simulink model "UAclient"  (R2019b)
settings: Solver=ode1  StartTime=0.0  StopTime=70  FixedStep=0.001  RelTol=1e-3
undefined symbols (not defined in the file or in its folder): sigbuilder_block
settings Model: Creator=y0n  LastModifiedBy=y0n
settings DataIOCC: SaveOutput=off  SignalLogging=off  DSMLogging=off  SaveTime=off  ReturnWorkspaceOutputsName=VehicleOut
settings DebuggingCC: AlgebraicLoopMsg=none  UnderSpecifiedDimensionMsg=error
settings SFSimCC: CustomCodeUndefinedFunction=UseInterfaceOnly

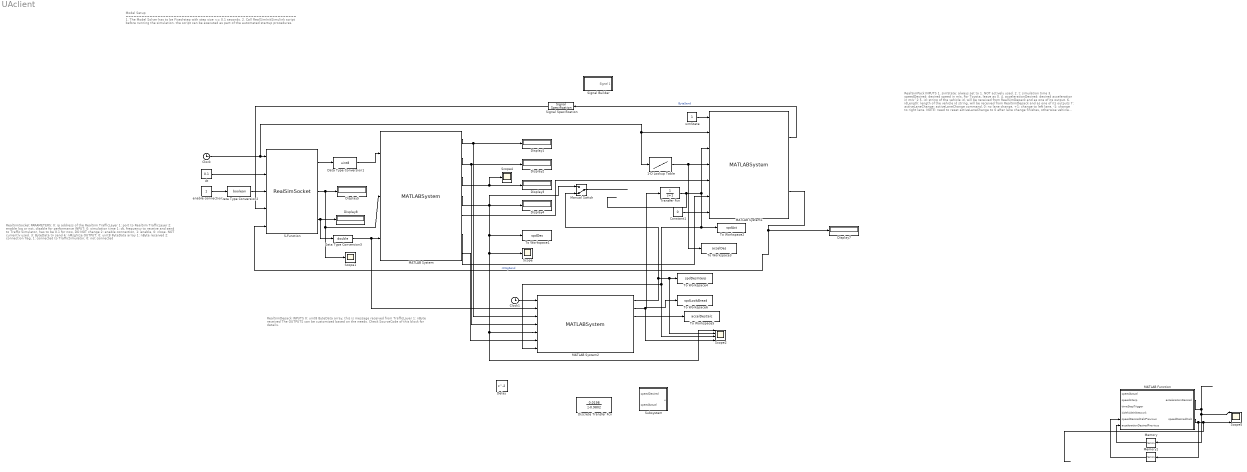
== system UAclient ==
  note: Model Setup
      | ================================================================
      | 1. The Model Solver has to be Fixed-step with step size <= 0.1 seconds.
      | 2. Call RealSimInitSimulink script before running the simulation. the script can be executed as part of the automated startup procedures.
  note: RealSimSocket
      | PARAMETERS:
      | 0: ip address of the RealSim TrafficLayer
      | 1: port to RealSim TrafficLayer
      | 2: enable log or not, disable for performance
      | INPUT:
      | 0: simulation time
      | 1: dt, frequency to receive and send to Traffic Simulator, has to be 0.1 for now, DO NOT change
      | 2: enable connection, 1: enable, 0: close. NOT currently used.
      | 3: ByteData to send
      | 4: nMsgSize
      |
      | OUTPUT:
      | 0: uint8 ByteData array
      | 1: nByte received
      | 2: connection flag, 1: connected to TrafficSimulator, 0: not connected
  note: RealSimPack
      | INPUTS
      | 1. simState: always set to 1. NOT actively used.
      | 2. t: simulation time
      | 3. speedDesired: desired speed in m/s, For Toyota, leave as 0.
      | 4. accelerationDesired: desired acceleration in m/s^2
      | 5. id: string of the vehicle id, will be received from RealSimDepack and as one of its output.
      | 6. idLength: length of the vehicle id string, will be received from RealSimDepack and as one of its outputs
      | 7: activeLaneChange: activeLaneChange command, 0: no lane change, +1: change to left lane, -1: change to right lane. NOTE: need to reset activeLaneChange to 0 after lane change finishes, otherwise vehicle will keep making lane change. Will receive 0 activeLaneChangeFdbk from RealSimDepack when lane change finishes.
      |
      | NOTE 1: Currently, only speedDesired and/or accelerationDesired can be sent to VISSIM/SUMO. The data format receive and send are the same so other mesage fields of the send data are irrelevant and can be set to empty or zero.
      |
      | NOTE 2: if select both speedDesired and accelerationDesired
      | in config.yaml, then only accelerationDesired will be used
      | to control vehicles in TrafficSimulator. if only one of
      | speedDesired and accelerationDesired selected in
      | config.yaml, then the one selected will be used for
      | control, the other input can be leave as 0.
      |
      | NOTE 3: for VISSIM, speedDesired or accelerationDesired will be the control command 0.2 seconds in the future.
      |
      | OUTPUTS
      | 1.ByteData: bytes vector that will be sent to TrafficSimualtor
      | 2.nMsgSize: size of bytes to be sent
  note: RealSimDepack
      | INPUTS
      | 0: uint8 ByteData array, this is message received from TrafficLayer
      | 1: nByte received
      |
      | The OUTPUTS can be customized based on the needs. Check SourceCode of this block for details.
  1-D Lookup Table : Lookup_n-D  NumberOfTableDimensions=1  BreakpointsForDimension1=[0 20 20.001 30 40 50 60 70 80 90 100]  Table=[0 0 0.2 0.2 -0.2 0.1 -0.1 0.3 -0.3 0 0 ]  InternalRulePriority=Speed  RndMeth=Simplest  InputSameDT=on
  Clock : Clock
  Clock1 : Clock
  Constant1 : Constant  Value=0
  Data Type Conversion1 : DataTypeConversion  OutDataTypeStr=uint8
  Data Type Conversion2 : DataTypeConversion  OutDataTypeStr=boolean
  Data Type Conversion3 : DataTypeConversion  OutDataTypeStr=double
  Delay : Delay
  Discrete Transfer Fcn : DiscreteTransferFcn  Numerator=[0.0198]  Denominator=[1 -0.9802]
  Display{1..5,7..8} (7 alike) : Display
  MATLAB Function : MATLAB Function  TreatAsAtomicUnit=on
  MATLAB System : MATLABSystem  System=RealSimDepack  VehicleMessageFieldDefInputVec=VehicleMessageFieldDefInputVec  SimulateUsing=Code generation
      mask Type: RealSimDepack
      mask Display:
      | disp('RealSimDepack');
      | port_label('input',1,'ByteData');
      | port_label('input',2,'nByte');
      | port_label('input',3,'connectionState');
      | port_label('output',1,'simState');
      | port_label('output',2,'t');
      | port_label('output',3,'nVeh');
      | port_label('output',4,'speed');
      | port_label('output',5,'id');
      | port_label('output',6,'idLen');
      | port_label('output',7,'isVehicleInNetwork');
  MATLAB System1 : MATLABSystem  System=RealSimPack  VehicleMessageFieldDefInputVec=VehicleMessageFieldDefInputVec  SimulateUsing=Code generation
      mask Type: RealSimPack
      mask Display:
      | disp('RealSimPack');
      | port_label('input',1,'simState');
      | port_label('input',2,'t');
      | port_label('input',3,'speedDesired');
      | port_label('input',4,'accelerationDesired');
      | port_label('input',5,'id');
      | port_label('input',6,'idLength');
      | port_label('input',7,'activeLaneChange');
      | port_label('output',1,'ByteData');
      | port_label('output',2,'nMsgSize');
  MATLAB System2 : MATLABSystem  System=RealSimInterpSpeed  initialSpeed=15.7  speedInterpolationMode=0  speedLookAheadHorizon=1  speedUpperBound=20  SimulateUsing=Code generation
      mask Type: RealSimInterpSpeed
      mask Display:
      | disp('RealSimInterpSpeed');
      | port_label('input',1,'simulationTime');
      | port_label('input',2,'connectionState');
      | port_label('input',3,'simState');
      | port_label('input',4,'timeReceive');
      | port_label('input',5,'speedReceive');
      | port_label('input',6,'isVehicleInNetwork');
      | port_label('input',7,'speedActual');
      | port_label('output',1,'speedInterp');
      | port_label('output',2,'speedLookAhead');
      | port_label('output',3,'accelerationDesired');
      | port_label('output',4,'timeSimulator');
      | port_label('output',5,'timeStepSimulator');
      | port_label('output',6,'timeStepTrigger');
      | port_label('output',7,'RealSimDelay');
  Manual Switch : ManualSwitch  CurrentSetting=0
  Memory : Memory
  Memory1 : Memory
  S-Function : S-Function  FunctionName=RealSimSocket  Parameters='127.0.0.1', 2333, 0  SFunctionDeploymentMode=off  EnableBusSupport=off
  Scope : Scope
  Scope1 : Scope
  Scope2 : Scope  NumInputPorts=4
  Scope4 : Scope
  Scope5 : Scope  NumInputPorts=4
  Signal Builder : Subsystem  Tag=STV Subsys  LoadFcn=sigbuilder_block('load');  StartFcn=sigbuilder_block('start');  StopFcn=sigbuilder_block('stop');  ClipboardFcn=sigbuilder_block('clipboard');  mask(Sigbuilder block){tuvar=[0:10]}
      mask help: Simulink:masks:SigbuilderBlock_MD
      mask init:
      | if ~strcmp(get_param(bdroot(gcbh),'SimulationStatus'),'stopped') tuvar = sigbuilder_block('maskInit'); end
      settings: CopyFcn=sigbuilder_block('copy');  DeleteFcn=sigbuilder_block('delete');  ModelCloseFcn=sigbuilder_block('modelClose');  PreSaveFcn=sigbuilder_block('preSave');  PauseFcn=sigbuilder_block('pause');  ContinueFcn=sigbuilder_block('continue');  NameChangeFcn=sigbuilder_block('namechange');  OpenFcn=sigbuilder_block('open',[6 30 1428 771.75 ]);  CloseFcn=sigbuilder_block('close');
      mask Display: plot(0, 0, 100, 100,[2, 2, 32, 32, 2], [68, 8, 8, 68, 68],[32, 2], [38, 38], [32, 19, 2],[53, 60, 44], [32, 17, 17, 2],[16, 16, 31, 31]);txt = getActiveGroup(gcbh);text(2, 100, txt,'verticalAlignment', 'top');
  Signal Specification : SignalSpecification  Dimensions=[200 1]
  Subsystem : Subsystem
  To Workspace1 : ToWorkspace  VariableName=spdDes  SaveFormat=Structure With Time  SampleTime=-1
  To Workspace2 : ToWorkspace  VariableName=spdAct  SaveFormat=Structure With Time  SampleTime=-1
  To Workspace3 : ToWorkspace  VariableName=accelDes  SaveFormat=Structure With Time  SampleTime=-1
  To Workspace4 : ToWorkspace  VariableName=spdDesInterp  SaveFormat=Structure With Time  SampleTime=-1
  To Workspace5 : ToWorkspace  VariableName=accelDesCalc  SaveFormat=Structure With Time  SampleTime=-1
  To Workspace6 : ToWorkspace  VariableName=spdLookAhead  SaveFormat=Structure With Time  SampleTime=-1
  Transfer Fcn : TransferFcn  Denominator=[1 1]
  dt : Constant  Value=0.1
  enable connection : Constant
  simState : Constant
  wires:
  Clock/1 -> MATLAB System1/2, 1-D Lookup Table/1, S-Function/1
  dt/1 -> S-Function/2
  simState/1 -> MATLAB System1/1
  MATLAB System1/1 -> Signal Specification/1  "ByteSend"
  MATLAB System1/2 -> S-Function/5, Display7/1  "nMsgSend"
  S-Function/1 -> Data Type Conversion1/1
  S-Function/2 -> Scope1/1, MATLAB System/2, Display5/1
  Data Type Conversion1/1 -> MATLAB System/1
  enable connection/1 -> Data Type Conversion2/1
  Data Type Conversion2/1 -> S-Function/3
  MATLAB System/1 -> Display1/1, MATLAB System2/3
  Constant1/1 -> MATLAB System1/7
  Signal Specification/1 -> S-Function/4
  1-D Lookup Table/1 -> To Workspace3/1, MATLAB System1/4
  MATLAB System/3 -> Scope4/1, Display3/1
  S-Function/3 -> Data Type Conversion3/1, Display8/1
  MATLAB System/5 -> MATLAB System1/5
  MATLAB System/6 -> MATLAB System1/6
  Transfer Fcn/1 -> MATLAB System1/3, To Workspace2/1, Scope2/3, MATLAB System2/7
  MATLAB System2/1 -> Manual Switch/2, Scope2/2, To Workspace4/1
  Clock1/1 -> MATLAB System2/1
  MATLAB System/7 -> MATLAB System2/6
  Data Type Conversion3/1 -> MATLAB System/3, MATLAB System2/2
  MATLAB System/4 -> Manual Switch/1, To Workspace1/1, MATLAB System2/5, Scope2/1, Scope/1, Display4/1
  MATLAB System/2 -> MATLAB System2/4, Display2/1
  Manual Switch/1 -> ?
  MATLAB System2/2 -> To Workspace6/1, Scope2/4, Transfer Fcn/1
  MATLAB System2/3 -> To Workspace5/1
  ? -> Scope5/3
  Memory1/1 -> MATLAB Function/5(speedDesiredCalcPrevious)
  Memory/1 -> MATLAB Function/6(accelerationDesiredPrevious)
  ? -> MATLAB Function/4(isVehicleInNetwork)
  ? -> MATLAB Function/3(timeStepTrigger)
  ? -> Scope5/2
  MATLAB Function/1(accelerationDesired) -> Scope5/1, Memory/1
  MATLAB Function/2(speedDesiredCalc) -> Scope5/4, Memory1/1
  ? -> MATLAB Function/1(speedActual)
  ? -> MATLAB Function/2(speedInterp)

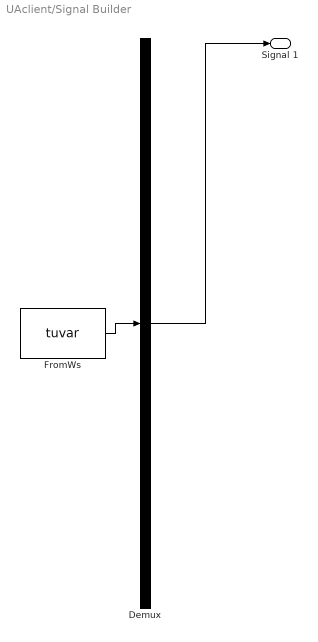
== system UAclient/Signal Builder ==
  Demux : Demux  Tag=STV Demux  Outputs=1
  FromWs : FromWorkspace  Tag=STV FromWs  VariableName=tuvar  SampleTime=0
      SigBuilderData=|
      | common.afterFinalStr = 'Extrapolate'
      | common.sampleTime = 0
      | dataSet.timeRange = [0 200]
      | dataSet.name = 'Group 1'
      | sbobj.Groups.Name = 'Group 1'
      | sbobj.Groups.Signals.Name = 'Signal 1'
      | sbobj.Groups.Signals.XData = [0 0.1 0.2 0.3 0.4 0.5 0.6 0.7 0.8 0.9 1 1.1 ... (2001 elements, 1x2001)]
      | sbobj.Groups.Signals.YData = [13 13 13 13 13 13 13 13 13 13 13 13 ... (2001 elements, 1x2001)]
      | sbobj.Groups.TimeRange = [0 200]
  Signal 1 : Outport  Tag=STV Outport  VectorParamsAs1DForOutWhenUnconnected=off
  wires:
  Demux/1 -> Signal 1/1
  FromWs/1 -> Demux/1

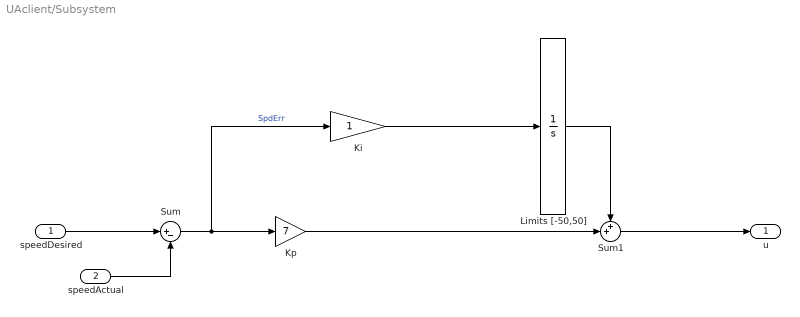
== system UAclient/Subsystem ==
  speedDesired : Inport
  speedActual : Inport  Port=2
  Ki : Gain
  Kp : Gain  Gain=7
  Limits [-50,50] : Integrator  LimitOutput=on  UpperSaturationLimit=50  LowerSaturationLimit=-50
  Sum : Sum  Inputs=|+-
  Sum1 : Sum  Inputs=++|
  u : Outport
  wires:
  Limits [-50,50]/1 -> Sum1/1
  Kp/1 -> Sum1/2
  Sum/1 -> Kp/1, Ki/1  "SpdErr"
  Sum1/1 -> u/1
  Ki/1 -> Limits [-50,50]/1
  speedActual/1 -> Sum/2
  speedDesired/1 -> Sum/1

== matlab function UAclient/MATLAB Function ==
  data: speedActual input; accelerationDesired output; speedInterp input; timeStepTrigger input; isVehicleInNetwork input; speedDesiredCalcPrevious input; accelerationDesiredPrevious input; speedDesiredCalc output
function [accelerationDesired, speedDesiredCalc] = fcn(speedActual, speedInterp, timeStepTrigger, isVehicleInNetwork, speedDesiredCalcPrevious, accelerationDesiredPrevious)

if isVehicleInNetwork
    if timeStepTrigger == 1
        % speedInterp is from SUMO, speedActual
        accelerationDesired = (speedInterp-speedActual)/0.1;
        speedDesiredCalc = min(max(0, speedActual + 10*0.1*accelerationDesired), 20);
    else
        accelerationDesired = accelerationDesiredPrevious;
        speedDesiredCalc = speedDesiredCalcPrevious;
    end
else
    accelerationDesired = 0;
    speedDesiredCalc = speedInterp;
end
